simulink model "Single_Phase_Grid_Connected_Inverter_With_PV_System_Final"  (R2023b)
settings: Solver=ode45  StartTime=0.0  StopTime=0.5  FixedStep=1e-6  MaxStep=1e-7  MinStep=1e-8  RelTol=1e-3
libraries: spsSeriesRLCBranchLib x8, spsCurrentMeasurementLib x6, spsIGBTDiodeLib x5, spsVoltageMeasurementLib x3, spsFirstOrderFilterLib x2, slpidlib x2, spsAlphaBetaZerotodq0Lib x1, simulink x1, spsDiodeLib x1, spsPVArrayLib x1, spsPWMGeneratorDCDCLib x1, spsPowerPhasorLib x1
settings Model: Creator=aoni5  LastModifiedBy=aoni5

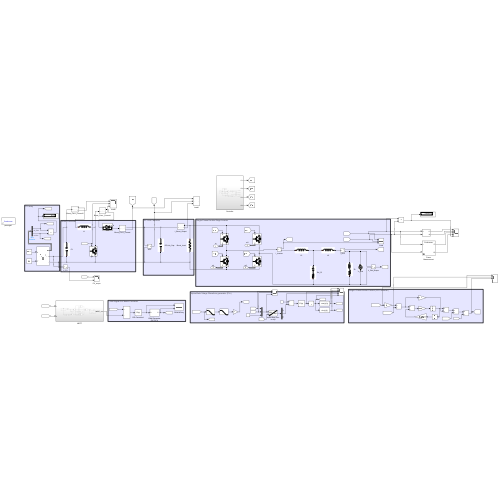
[thumbnail: Simulink's stored preview of the top-level diagram]
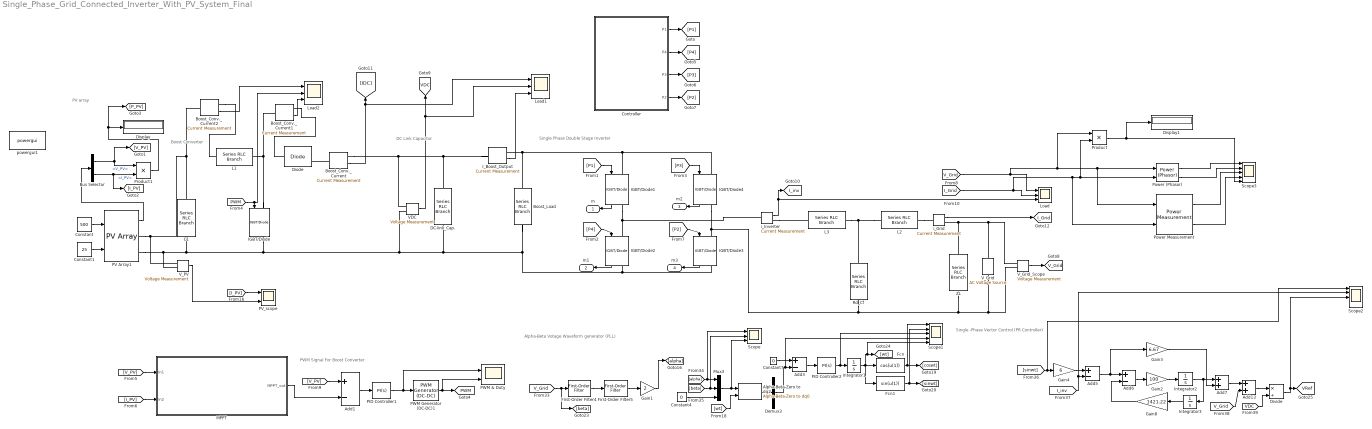
== system Single_Phase_Grid_Connected_Inverter_With_PV_System_Final ==
  note: Single -Phase Vector Control (PR Controller)
  note: Single Phase Double Stage Inverter
  note: DC Link Capacitor
  note: PWM Signal For Boost Converter
  note: PV array
  note: Boost Converter
  note: Alpha-Beta Votage Waveform generator (PLL)
  Add{1,3,5..6} (4 alike) : Sum  Inputs=+-
  Add13 : Sum
  Add7 : Sum
  Alpha-Beta-Zero to dq2 : spsAlphaBetaZerotodq0Lib/Alpha-Beta-Zero to dq0  Alignment=90 degrees behind phase A axis
  Boost_Conv._Current : spsCurrentMeasurementLib/Current Measurement  PhasorSimulation=off  OutputType=Complex  PSBequivalent=0
  Boost_Conv._Current1 : spsCurrentMeasurementLib/Current Measurement  PhasorSimulation=off  OutputType=Complex  PSBequivalent=0
  Boost_Conv._Current2 : spsCurrentMeasurementLib/Current Measurement  PhasorSimulation=off  OutputType=Complex  PSBequivalent=0
  Boost_Load : spsSeriesRLCBranchLib/Series RLC Branch  LConnTagsString=__new0  RConnTagsString=__new0  BranchType=R  Resistance=5000  Inductance=1e-3  SetiL0=off  InitialCurrent=0  Capacitance=5000e-6  Setx0=off  InitialVoltage=0  Measurements=None
  Bus Selector : BusSelector  OutputSignals=V_PV,I_PV
  C1 : spsSeriesRLCBranchLib/Series RLC Branch  LConnTagsString=__new0  RConnTagsString=__new0  BranchType=C  Resistance=1e-3  Inductance=1e-3  SetiL0=off  InitialCurrent=0  Capacitance=500e-6  Setx0=off  InitialVoltage=400  Measurements=None
  Constant : Constant  Value=500
  Constant1 : Constant  Value=25
  Constant4 : Constant  Value=0
  Constant7 : Constant  Value=0
  Controller : Subsystem
  DC-link_Cap. : spsSeriesRLCBranchLib/Series RLC Branch  LConnTagsString=__new0  RConnTagsString=__new0  BranchType=C  Resistance=5.97  Inductance=1e-3  SetiL0=off  InitialCurrent=0  Capacitance=5500e-6  Setx0=off  InitialVoltage=0  Measurements=None
  Demux3 : Demux  Outputs=3
  Diode : spsDiodeLib/Diode  Ron=0.001  Lon=0  Vf=0.8  IC=0  UseSnubber=0  Rs=500  Cs=250e-9  Measurements=on
  Display : Display
  Display1 : Display
  Divide : Product  Inputs=*/
  Fcn : Fcn  Expr=cos(u(1))
  Fcn1 : Fcn  Expr=sin(u(1))
  First-Order Filter4 : spsFirstOrderFilterLib/First-Order Filter  FilterType=Lowpass  Tc=1/(2*pi*60)  Ts=0  Initialize=off  Vac_Init=[0, 0, 60]  Vdc_Init=0  PlotResponse=off  FreqRange="[0,  200,  1]"
  First-Order Filter5 : spsFirstOrderFilterLib/First-Order Filter  FilterType=Lowpass  Tc=1/(2*pi*60)  Ts=0  Initialize=off  Vac_Init=[0, 0, 60]  Vdc_Init=0  PlotResponse=off  FreqRange="[0,  200,  1]"
  Gain1 : Gain  Gain=2
  Gain2 : Gain  Gain=100
  Gain3 : Gain  Gain=6.67
  Gain4 : Gain  Gain=6
  Gain8 : Gain  Gain=1421.22
  IGBT/Diode{,1..4} (5 alike) : spsIGBTDiodeLib/IGBT//Diode  Ron=1e-3  Rs=1e5  Cs=inf  Measurements=on
  I_Boost_Output : spsCurrentMeasurementLib/Current Measurement  PhasorSimulation=off  OutputType=Complex  PSBequivalent=0
  Integrator1 : Integrator
  Integrator2 : Integrator
  Integrator3 : Integrator
  L1 : spsSeriesRLCBranchLib/Series RLC Branch  LConnTagsString=__new0  RConnTagsString=__new0  BranchType=L  Resistance=1e-3  Inductance=20e-3  SetiL0=off  InitialCurrent=0  Capacitance=1000e-6  Setx0=off  InitialVoltage=0  Measurements=None
  L2 : spsSeriesRLCBranchLib/Series RLC Branch  LConnTagsString=__new0  RConnTagsString=__new0  BranchType=L  Resistance=2.5  Inductance=250e-6  SetiL0=off  InitialCurrent=0  Capacitance=50e-6  Setx0=off  InitialVoltage=0  Measurements=None
  L3 : spsSeriesRLCBranchLib/Series RLC Branch  LConnTagsString=__new0  RConnTagsString=__new0  BranchType=L  Resistance=2.5  Inductance=1e-3  SetiL0=off  InitialCurrent=0  Capacitance=50e-6  Setx0=off  InitialVoltage=0  Measurements=None
  Load : Scope  NumInputPorts=3
  Load1 : Scope  NumInputPorts=3
  Load2 : Scope  NumInputPorts=3
  MPPT : Subsystem
  Mux3 : Mux  Inputs=3
  PID Controller1 : slpidlib/PID Controller  Controller=PI  Form=Parallel  TimeDomain=Continuous-time  UseExternalTs=off  SampleTime=-1  IntegratorMethod=Forward Euler  FilterMethod=Forward Euler  ControllerParametersSource=internal  P=1  I=1  UseKiTs=off  D=0  N=100  UseFilter=on  TunerSelectOption=Transfer Function Based (PID Tuner App)  InitialConditionSource=internal  InitialConditionForIntegrator=0  InitialConditionForFilter=0  DifferentiatorICPrevScaledInput=0  ExternalReset=none  TrackingMode=off  Kt=1  LimitOutput=off  SatLimitsSource=internal  UpperSaturationLimit=inf  LowerSaturationLimit=-inf  LinearizeAsGain=on  AntiWindupMode=none  Kb=1  LimitIntegrator=off  UpperIntegratorSaturationLimit=inf  LowerIntegratorSaturationLimit=-inf  POutMin=[]  POutMax=[]  IOutMin=[]  IOutMax=[]  DOutMin=[]  DOutMax=[]  NOutMin=[]  NOutMax=[]  SumOutMin=[]  SumOutMax=[]  SaturationOutMin=[]  SaturationOutMax=[]  PParamMin=[]  PParamMax=[]  IParamMin=[]  IParamMax=[]  DParamMin=[]  DParamMax=[]  NParamMin=[]  NParamMax=[]  KbParamMin=[]  KbParamMax=[]  KtParamMin=[]  KtParamMax=[]  KbOutMin=[]  KbOutMax=[]  KtOutMin=[]  KtOutMax=[]  IntegratorOutMin=[]  IntegratorOutMax=[]  FilterOutMin=[]  FilterOutMax=[]  SumI1OutMin=[]  SumI1OutMax=[]  SumI2OutMin=[]  SumI2OutMax=[]  SumI3OutMin=[]  SumI3OutMax=[]  SumI4OutMin=[]  SumI4OutMax=[]  SumDOutMin=[]  SumDOutMax=[]  DifferentiatorOutMin=[]  DifferentiatorOutMax=[]  FilterDiffOutCoefMin=[]  FilterDiffOutCoefMax=[]  ReciprocalOutMin=[]  ReciprocalOutMax=[]  SumDenOutMin=[]  SumDenOutMax=[]  SumNumOutMin=[]  SumNumOutMax=[]  DivideOutMin=[]  DivideOutMax=[]  UdiffTsProdOutMin=[]  UdiffTsProdOutMax=[]  NTsProdOutMin=[]  NTsProdOutMax=[]  UintegralTsProdOutMin=[]  UintegralTsProdOutMax=[]  UngainTsProdOutMin=[]  UngainTsProdOutMax=[]  ClampingZeroOutDataTypeStr=Inherit: Inherit via back propagation  ClampingZeroOutMin=[]  ClampingZeroOutMax=[]  FilterDenConstantOutDataTypeStr=Inherit: Inherit via back propagation  FilterDenConstantOutMin=[]  FilterDenConstantOutMax=[]  PCopyOutDataTypeStr=Inherit: Inherit via back propagation  PCopyOutMin=[]  PCopyOutMax=[]  NCopyOutDataTypeStr=Inherit: Inherit via back propagation  NCopyOutMin=[]  NCopyOutMax=[]  IntegratorContinuousStateAttributes=''  IntegratorStateMustResolveToSignalObject=off  IntegratorRTWStateStorageClass=Auto  FilterContinuousStateAttributes=''  FilterStateMustResolveToSignalObject=off  FilterRTWStateStorageClass=Auto  ParallelPVariant=InternalParameters  IdealPVariant=Disabled  IVariant=InternalParameters  DVariant=Disabled  IntegratorVariant=Continuous  SatVariant=Disabled  AWVariant=Passthrough  PCopyVariant=Disabled  TRVariant=Disabled  FdbkBlocksVariant=Forward  IdealPFdbkVariant=Disabled  SatFdbkVariant=Disabled  DerivativeFilterVariant=Disabled  NVariant=Disabled  NCopyVariant=Disabled_SignalSpec  FilterICVariant=Disabled  IntegratorICVariant=InternalICs  ExternalResetVariant=Disabled  TRSumVariant=Passthrough  SumFdbkVariant=Disabled  SumVariant=Sum_PI  TsampFilterVariant=InternalTs  TsampNgainVariant=Passthrough  TsampIntegralVariant=Disabled_SignalSpec  ExternalSaturationOutDataTypeStr=Inherit: Same as second input
  PID Controller2 : slpidlib/PID Controller  Controller=PI  Form=Parallel  TimeDomain=Continuous-time  UseExternalTs=off  SampleTime=-1  IntegratorMethod=Forward Euler  FilterMethod=Forward Euler  ControllerParametersSource=internal  P=10  I=50000  UseKiTs=off  D=0  N=100  UseFilter=on  TunerSelectOption=Transfer Function Based (PID Tuner App)  InitialConditionSource=internal  InitialConditionForIntegrator=0  InitialConditionForFilter=0  DifferentiatorICPrevScaledInput=0  ExternalReset=none  TrackingMode=off  Kt=1  LimitOutput=off  SatLimitsSource=internal  UpperSaturationLimit=inf  LowerSaturationLimit=-inf  LinearizeAsGain=on  AntiWindupMode=none  Kb=1  LimitIntegrator=off  UpperIntegratorSaturationLimit=inf  LowerIntegratorSaturationLimit=-inf  POutMin=[]  POutMax=[]  IOutMin=[]  IOutMax=[]  DOutMin=[]  DOutMax=[]  NOutMin=[]  NOutMax=[]  SumOutMin=[]  SumOutMax=[]  SaturationOutMin=[]  SaturationOutMax=[]  PParamMin=[]  PParamMax=[]  IParamMin=[]  IParamMax=[]  DParamMin=[]  DParamMax=[]  NParamMin=[]  NParamMax=[]  KbParamMin=[]  KbParamMax=[]  KtParamMin=[]  KtParamMax=[]  KbOutMin=[]  KbOutMax=[]  KtOutMin=[]  KtOutMax=[]  IntegratorOutMin=[]  IntegratorOutMax=[]  FilterOutMin=[]  FilterOutMax=[]  SumI1OutMin=[]  SumI1OutMax=[]  SumI2OutMin=[]  SumI2OutMax=[]  SumI3OutMin=[]  SumI3OutMax=[]  SumI4OutMin=[]  SumI4OutMax=[]  SumDOutMin=[]  SumDOutMax=[]  DifferentiatorOutMin=[]  DifferentiatorOutMax=[]  FilterDiffOutCoefMin=[]  FilterDiffOutCoefMax=[]  ReciprocalOutMin=[]  ReciprocalOutMax=[]  SumDenOutMin=[]  SumDenOutMax=[]  SumNumOutMin=[]  SumNumOutMax=[]  DivideOutMin=[]  DivideOutMax=[]  UdiffTsProdOutMin=[]  UdiffTsProdOutMax=[]  NTsProdOutMin=[]  NTsProdOutMax=[]  UintegralTsProdOutMin=[]  UintegralTsProdOutMax=[]  UngainTsProdOutMin=[]  UngainTsProdOutMax=[]  ClampingZeroOutDataTypeStr=Inherit: Inherit via back propagation  ClampingZeroOutMin=[]  ClampingZeroOutMax=[]  FilterDenConstantOutDataTypeStr=Inherit: Inherit via back propagation  FilterDenConstantOutMin=[]  FilterDenConstantOutMax=[]  PCopyOutDataTypeStr=Inherit: Inherit via back propagation  PCopyOutMin=[]  PCopyOutMax=[]  NCopyOutDataTypeStr=Inherit: Inherit via back propagation  NCopyOutMin=[]  NCopyOutMax=[]  IntegratorContinuousStateAttributes=''  IntegratorStateMustResolveToSignalObject=off  IntegratorRTWStateStorageClass=Auto  FilterContinuousStateAttributes=''  FilterStateMustResolveToSignalObject=off  FilterRTWStateStorageClass=Auto  ParallelPVariant=InternalParameters  IdealPVariant=Disabled  IVariant=InternalParameters  DVariant=Disabled  IntegratorVariant=Continuous  SatVariant=Disabled  AWVariant=Passthrough  PCopyVariant=Disabled  TRVariant=Disabled  FdbkBlocksVariant=Forward  IdealPFdbkVariant=Disabled  SatFdbkVariant=Disabled  DerivativeFilterVariant=Disabled  NVariant=Disabled  NCopyVariant=Disabled_SignalSpec  FilterICVariant=Disabled  IntegratorICVariant=InternalICs  ExternalResetVariant=Disabled  TRSumVariant=Passthrough  SumFdbkVariant=Disabled  SumVariant=Sum_PI  TsampFilterVariant=InternalTs  TsampNgainVariant=Passthrough  TsampIntegralVariant=Disabled_SignalSpec  ExternalSaturationOutDataTypeStr=Inherit: Same as second input
  PV Array1 : spsPVArrayLib/PV Array  Npar=2  Nser=3  PlotType=array @ 25 deg.C & specified irradiances  S_vec=[ 1000 800 600 400 200]  Temp_C_vec="[ 25  ]"  ModuleName=User-defined  PlotWhenSelected=off  Pm=314.1504  Ncell=81  Voc=81*0.727  Isc=6.45  Vm=0.640*81  Im=6.06  beta_Voc_pc=-1.74e-3/0.727*100  alpha_Isc_pc=2.9e-3/6.45*100  beta_Voc=-0.14094  alpha_Isc=0.0029  IL=6.4513  I0=1.3343e-12  nI=0.96977  Rsh=326.9714  Rs=0.064206  RobustModel=off  RobustCellTemperature=313.3991  BAL=on  Tc=1e-6  Tfilter=5e-5
  PV_scope : Scope  NumInputPorts=2
  PWM & Duty : Scope  NumInputPorts=2
  PWM Generator (DC-DC)1 : spsPWMGeneratorDCDCLib/PWM Generator (DC-DC)  Fsw=7000  Ts=1e-6
  Power (Phasor) : spsPowerPhasorLib/Power (Phasor)
      settings: LibrarySourceBlock=|
      | sps_lib/Sensors and Measurements/Power
      | (Phasor)
  Power Measurement : eePowerMeasurement/Power Measurement  LabelModeActiveChoice=Continuous  F=60  K=[0 1 2 3]  Ts=0
  Product : Product
  Product1 : Product
  Rd_Cf : spsSeriesRLCBranchLib/Series RLC Branch  LConnTagsString=__new0  RConnTagsString=__new0  BranchType=RC  Resistance=5.97  Inductance=1e-3  SetiL0=off  InitialCurrent=0  Capacitance=5.6e-6  Setx0=off  InitialVoltage=0  Measurements=None
  Scope : Scope  NumInputPorts=3
  Scope1 : Scope  NumInputPorts=5
  Scope2 : Scope  NumInputPorts=5
  Scope3 : Scope  NumInputPorts=5
  VDC : spsVoltageMeasurementLib/Voltage Measurement  PhasorSimulation=off  OutputType=Complex  PSBequivalent=0
  V_Grid : spsACVoltageSourceLib/AC Voltage Source  Amplitude=300  Phase=0  Frequency=60  SampleTime=0  Measurements=None  BusType=swing  Pref=10e3  Qref=0  Qmin=-inf  Qmax=+inf
  V_Grid_Scope : spsVoltageMeasurementLib/Voltage Measurement  PhasorSimulation=off  OutputType=Complex  PSBequivalent=0
  V_PV : spsVoltageMeasurementLib/Voltage Measurement  PhasorSimulation=off  OutputType=Complex  PSBequivalent=0
  ZL : spsSeriesRLCBranchLib/Series RLC Branch  LConnTagsString=__new0  RConnTagsString=__new0  BranchType=RL  Resistance=5  Inductance=5e-3  SetiL0=off  InitialCurrent=0  Capacitance=1e-6  Setx0=off  InitialVoltage=0  Measurements=None
  i_Grid : spsCurrentMeasurementLib/Current Measurement  PhasorSimulation=off  OutputType=Complex  PSBequivalent=0
  i_Inverter : spsCurrentMeasurementLib/Current Measurement  PhasorSimulation=off  OutputType=Complex  PSBequivalent=0
  powergui1 : sps_lib/powergui  Priority=1  SimulationMode=Continuous  SampleTime=50e-6  frequency=60  Iterations=50  frequencyindice=0  Pbase=100e6  ErrMax=1e-4  UnitsV=kV  UnitsW=MW  buscounter=0  FunctionMessages=off  echomessages=off  EnableUseOfTLC=off  CurrentSourceSwitches=off  DisableSnubberDevices=off  DisableRonSwitches=off  DisableVfSwitches=off  DisplayEquations=off  AutomaticDiscreteSolvers=off  SolverType=Tustin/Backward Euler (TBE)  Interpol=off  ExternalGateDelay=off  methode=off  Ts=100  x0status=blocks  SPID=on  SwTol=0  HookPort=off  NonlinearTolerance=1e-4  nMaxIteration=100  ContinueOnMaxIteration=off  RestoreLinks=warning  ResistiveCurrentMeasurement=off  Frange=[0:2:500]  Ylog=off  Xlog=on  ShowGrid=off  save=off  variable=ZData  structure=0  ZoomFFT=off  StartTime=0.0  cycles=1  DisplayStyle=1  fundamental=60  FreqAxis=off  MaxFrequency=1000  frequencyindicesteady=1  RmsSteady=1  display=off
  m : Outport
  m1 : Outport  Port=2
  m2 : Outport  Port=3
  m3 : Outport  Port=4
  tag scope: I_Grid=global, I_inv=global, PWM=global, VDC=global, VRef=global, V_Grid=global
  wires:
  V_PV/1 -> PV_scope/2
  Constant/1 -> PV Array1/1
  Constant1/1 -> PV Array1/2
  Bus Selector/1 -> Product1/1, [V_PV]  "<V_PV>"
  PV Array1/1 -> Bus Selector/1
  [PWM] -> Load2/2, IGBT/Diode/1
  VDC/1 -> [VDC], Load1/2
  Product1/1 -> [P_PV], Display/1
  Boost_Conv._Current/1 -> Load1/1, [IDC]
  Bus Selector/2 -> Product1/2, [I_PV]  "<I_PV>"
  [I_PV] -> PV_scope/1
  [V_PV] -> MPPT/1(In1)
  [I_PV] -> MPPT/2(In2)
  PID Controller1/1 -> PWM & Duty/1, PWM Generator (DC-DC)1/1
  PWM Generator (DC-DC)1/1 -> PWM & Duty/2, [PWM]
  MPPT/1(MPPT_out) -> Add1/2
  Add1/1 -> PID Controller1/1
  [V_PV] -> Add1/1
  IGBT/Diode4/1 -> m2/1
  IGBT/Diode3/1 -> m3/1
  IGBT/Diode2/1 -> m1/1
  IGBT/Diode1/1 -> m/1
  Controller/4(P2) -> [P2]
  Controller/1(P1) -> [P1]
  Controller/3(P3) -> [P3]
  Controller/2(P4) -> [P4]
  [V_Grid] -> Product/1, Power Measurement/1, Power (Phasor)/1, Load/1
  i_Grid/1 -> [I_Grid]
  V_Grid_Scope/1 -> [V_Grid]
  i_Inverter/1 -> [I_inv], Load/3
  [P2] -> IGBT/Diode3/1
  [P4] -> IGBT/Diode2/1
  [P1] -> IGBT/Diode1/1
  [P3] -> IGBT/Diode4/1
  [I_Grid] -> Power Measurement/2, Product/2, Power (Phasor)/2, Load/2
  I_Boost_Output/1 -> Load1/3
  [wt] -> Alpha-Beta-Zero to dq2/2
  [alpha] -> Scope/1, Mux3/1
  Constant7/1 -> Add3/1
  Integrator1/1 -> Fcn1/1, Fcn/1, Scope1/5, [wt]
  Add3/1 -> PID Controller2/1
  Fcn/1 -> Scope1/1, [coswt]
  PID Controller2/1 -> Scope1/3, Integrator1/1
  [beta] -> Scope/2, Mux3/2
  Alpha-Beta-Zero to dq2/1 -> Demux3/1
  Constant4/1 -> Mux3/3
  First-Order Filter5/1 -> Gain1/1
  Gain1/1 -> [alpha]
  Mux3/1 -> Scope/3, Alpha-Beta-Zero to dq2/1
  [V_Grid] -> [beta], First-Order Filter4/1
  First-Order Filter4/1 -> First-Order Filter5/1
  Fcn1/1 -> Scope1/2, [sinwt]
  Integrator3/1 -> Gain8/1
  Gain2/1 -> Integrator2/1
  Divide/1 -> Scope2/3, [VRef]
  Integrator2/1 -> Add7/1, Integrator3/1
  [V_Grid] -> Add13/2
  Add7/1 -> Add13/1
  Gain3/1 -> Add7/2
  Gain8/1 -> Add6/2
  [I_inv] -> Scope2/2, Add5/2
  Add5/1 -> Gain3/1, Add6/1
  Gain4/1 -> Add5/1
  [sinwt] -> Scope2/1, Gain4/1
  Add6/1 -> Gain2/1
  Demux3/2 -> Scope1/4, Add3/2
  Boost_Conv._Current1/1 -> Load2/3
  Boost_Conv._Current2/1 -> Load2/1
  Power (Phasor)/1 -> Scope3/1
  Power (Phasor)/2 -> Scope3/2
  Power Measurement/1 -> Scope3/3
  Power Measurement/2 -> Scope3/4
  Product/1 -> Display1/1, Scope3/5
  [VDC] -> Divide/2
  Add13/1 -> Divide/1
  connections:
  IGBT/Diode/LConn1 -- Boost_Conv._Current1/LConn1 -- L1/RConn1
  Boost_Conv._Current/LConn1 -- Diode/RConn1
  V_PV/LConn1 -- PV Array1/RConn1 -- C1/RConn1 -- Boost_Conv._Current2/LConn1
  IGBT/Diode2/RConn1 -- Boost_Load/RConn1 -- PV Array1/RConn2 -- V_PV/LConn2 -- C1/LConn1 -- IGBT/Diode/RConn1 -- VDC/LConn2 -- DC-link_Cap./LConn1 -- IGBT/Diode3/RConn1
  VDC/LConn1 -- Boost_Conv._Current/RConn1 -- I_Boost_Output/LConn1 -- DC-link_Cap./RConn1
  L2/RConn1 -- i_Grid/LConn1
  i_Grid/RConn1 -- V_Grid_Scope/LConn1 -- V_Grid/RConn1 -- ZL/RConn1
  i_Inverter/RConn1 -- L3/LConn1
  IGBT/Diode1/RConn1 -- i_Inverter/LConn1 -- IGBT/Diode2/LConn1
  IGBT/Diode4/RConn1 -- V_Grid_Scope/LConn2 -- V_Grid/LConn1 -- ZL/LConn1 -- Rd_Cf/LConn1 -- IGBT/Diode3/LConn1
  L2/LConn1 -- Rd_Cf/RConn1 -- L3/RConn1
  Boost_Load/LConn1 -- I_Boost_Output/RConn1 -- IGBT/Diode1/LConn1 -- IGBT/Diode4/LConn1
  Boost_Conv._Current1/RConn1 -- Diode/LConn1
  Boost_Conv._Current2/RConn1 -- L1/LConn1

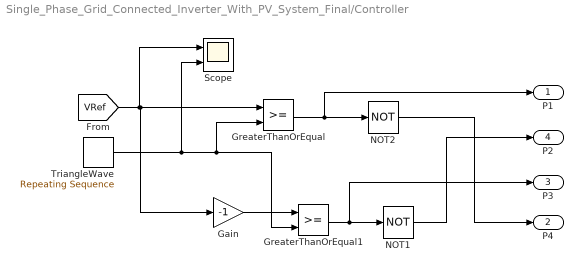
== system Single_Phase_Grid_Connected_Inverter_With_PV_System_Final/Controller ==
  Gain : Gain  Gain=-1
  GreaterThanOrEqual : RelationalOperator  OutDataTypeStr=boolean  RndMeth=Simplest  InputSameDT=off
  GreaterThanOrEqual1 : RelationalOperator  OutDataTypeStr=boolean  RndMeth=Simplest  InputSameDT=off
  NOT1 : Logic  Operator=NOT  IconShape=distinctive  AllPortsSameDT=off  OutDataTypeStr=boolean
  NOT2 : Logic  Operator=NOT  IconShape=distinctive  AllPortsSameDT=off  OutDataTypeStr=boolean
  Scope : Scope  NumInputPorts=2
  TriangleWave : simulink/Sources/Repeating Sequence  rep_seq_t=[0 50e-6 100e-6]  rep_seq_y=[-1 0 1]
  P1 : Outport
  P4 : Outport  Port=2
  P3 : Outport  Port=3
  P2 : Outport  Port=4
  wires:
  NOT1/1 -> P2/1
  GreaterThanOrEqual/1 -> P1/1, NOT2/1
  TriangleWave/1 -> GreaterThanOrEqual1/2, GreaterThanOrEqual/2, Scope/2
  Gain/1 -> GreaterThanOrEqual1/1
  GreaterThanOrEqual1/1 -> P3/1, NOT1/1
  NOT2/1 -> P4/1
  [VRef] -> Scope/1, Gain/1, GreaterThanOrEqual/1

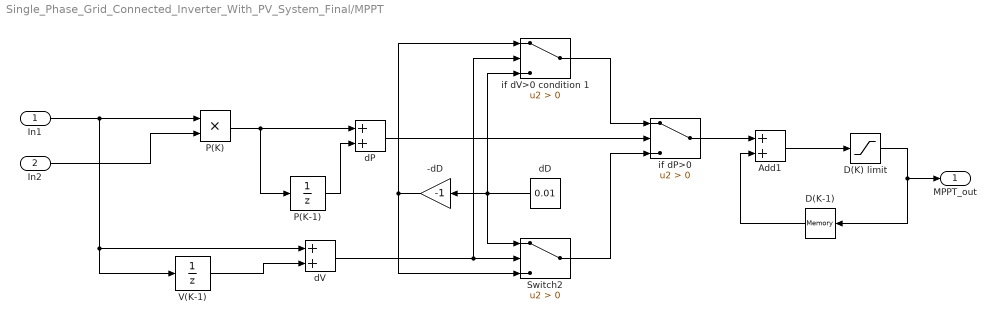
== system Single_Phase_Grid_Connected_Inverter_With_PV_System_Final/MPPT ==
  In1 : Inport
  In2 : Inport  Port=2
  -dD : Gain  Gain=-1
  Add1 : Sum
  D(K) limit : Saturate  UpperLimit=160  LowerLimit=145
  D(K-1) : Memory
  P(K) : Product
  P(K-1) : UnitDelay  SampleTime=-1  HasFrameUpgradeWarning=on
  Switch2 : Switch  Criteria=u2 > Threshold  SaturateOnIntegerOverflow=off  InputSameDT=off
  V(K-1) : UnitDelay  SampleTime=-1  HasFrameUpgradeWarning=on
  dD : Constant  Value=0.01
  dP : Sum
  dV : Sum
  if dP>0 : Switch  Criteria=u2 > Threshold  SaturateOnIntegerOverflow=off  InputSameDT=off
  if dV>0 condition 1 : Switch  Criteria=u2 > Threshold  SaturateOnIntegerOverflow=off  InputSameDT=off
  MPPT_out : Outport
  wires:
  D(K) limit/1 -> D(K-1)/1, MPPT_out/1
  -dD/1 -> if dV>0 condition 1/1, Switch2/3
  dP/1 -> if dP>0/2
  P(K-1)/1 -> dP/2
  dD/1 -> if dV>0 condition 1/3, Switch2/1, -dD/1
  Switch2/1 -> if dP>0/3
  D(K-1)/1 -> Add1/2
  if dP>0/1 -> Add1/1
  In1/1 -> V(K-1)/1, dV/1, P(K)/1
  Add1/1 -> D(K) limit/1
  dV/1 -> Switch2/2, if dV>0 condition 1/2
  if dV>0 condition 1/1 -> if dP>0/1
  V(K-1)/1 -> dV/2
  P(K)/1 -> dP/1, P(K-1)/1
  In2/1 -> P(K)/2
